simulink model "Model_SIR"  (R2023a)
settings: Solver=VariableStepAuto  StartTime=0.0  StopTime=100.0  RelTol=1e-3
model workspace (MAT data in the model file):
  b = 0.3
  g = 0.15
  n = 7700000
settings Model: Creator=joans  LastModifiedBy=joans
settings ModelReferenceCC: EnableRefExpFcnMdlSchedulingChecks=on

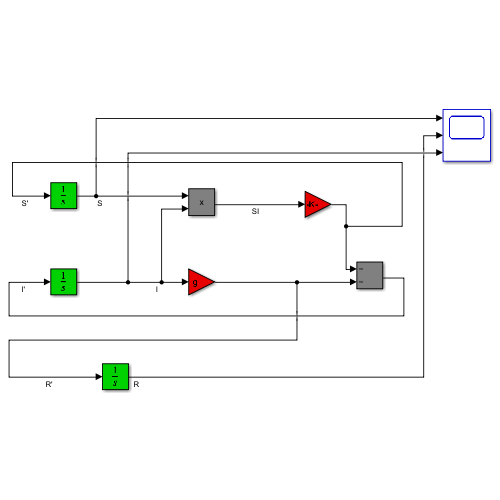
[thumbnail: Simulink's stored preview of the top-level diagram]
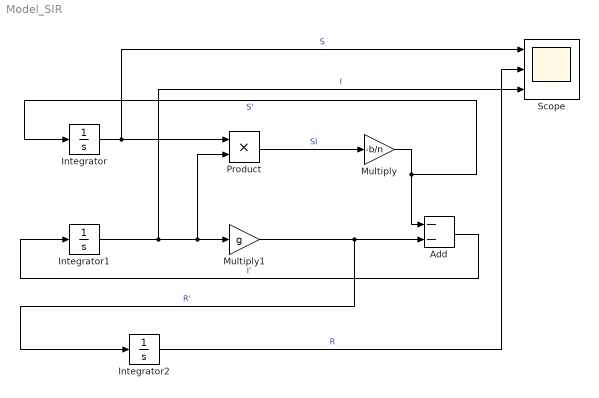
== system Model_SIR ==
  Add : Sum  Inputs=--
  Integrator : Integrator  InitialCondition=n
  Integrator1 : Integrator  InitialCondition=1000
  Integrator2 : Integrator
  Multiply : Gain  Gain=-b/n
  Multiply1 : Gain  Gain=g
  Product : Product
  Scope : Scope  NumInputPorts=3
  wires:
  Integrator/1 -> Product/1, Scope/1  "S"
  Integrator1/1 -> Scope/3, Product/2, Multiply1/1  "I"
  Product/1 -> Multiply/1  "SI"
  Multiply/1 -> Add/1, Integrator/1  "S'"
  Multiply1/1 -> Integrator2/1, Add/2  "R'"
  Add/1 -> Integrator1/1  "I'"
  Integrator2/1 -> Scope/2  "R"
